simulink model "MLC_Aero_Simulink"  (R2018a)
settings: Solver=ode1  StartTime=0.0  StopTime=50  FixedStep=0.002  RelTol=1e-3  EnableMultiTasking=on
values from neighbouring files (symbols this model uses):
  pitch_amp = pi/6    (= 0.523598775598)    [lqr_controller.m]
  pitch_freq = 0.4    [lqr_controller.m]
  yaw_amp = pi/4    (= 0.785398163397)    [lqr_controller.m]
  yaw_freq = 0.5    [lqr_controller.m]
undefined symbols (not defined in the file or in its folder): HIL, qc_get_step_size
libraries: quarc_library x18, cstblocks x5
settings Model: SimulationMode=external  ExtModeTrigDuration=20000  Creator=MLevis  LastModifiedBy=Student
settings SolverCC: PositivePriorityOrder=on
settings DataIOCC: LimitDataPoints=on  SaveFormat=Array
settings OptimizationCC: LifeSpan=inf
settings DebuggingCC: SolverPrmCheckMsg=warning  SFUnexpectedBacktrackingDiag=warning  SFNoUnconditionalDefaultTransitionDiag=warning  SFExecutionAtInitializationDiag=none
settings HardwareCC: ProdBitPerPointer=32  ProdBitPerSizeT=32  ProdBitPerPtrDiffT=32  ProdLargestAtomicFloat=None  ProdIntDivRoundTo=Undefined  ProdEndianess=Unspecified  ProdWordSize=32  ProdHWDeviceType=32-bit Generic
settings ModelReferenceCC: PropagateSignalLabelsOutOfModel=off
settings RTWCC: SystemTargetFile=quarc_win64.tlc  TemplateMakefile=quarc_default_tmf  Description=QUARC Win64 Target
settings CodeAppCC: StateflowObjectComments=on
settings STFCustomTargetCC: TargetPreCompLibLocation=C:\PROGRA~3\QUARC\lib\2018a\win64\release  ConcurrentExecutionCompliant=on  GeneratePreprocessorConditionals=Disable all  SystemTargetFile=quarc_win64.tlc
settings GRTTargetCC: TargetPreCompLibLocation=C:\PROGRA~3\QUARC\lib\2018a\win64\release  TargetLangStandard=C89/C90 (ANSI)  ParMdlRefBuildCompliant=off  CompOptLevelCompliant=off  GeneratePreprocessorConditionals=Disable all  CombineOutputUpdateFcns=off  MatFileLogging=off  CPPClassGenCompliant=off  GRTInterface=on  UseToolchainInfoCompliant=off  ExtMode=on  ExtModeMexFile=quarc_comm
settings ConfigComp: CovMetricSettings=dw  CovHtmlReporting=on  CovSaveCumulativeToWorkspaceVar=on  CovSaveSingleToWorkspaceVar=on  CovExternalEMLEnable=off  CovSFcnEnable=off

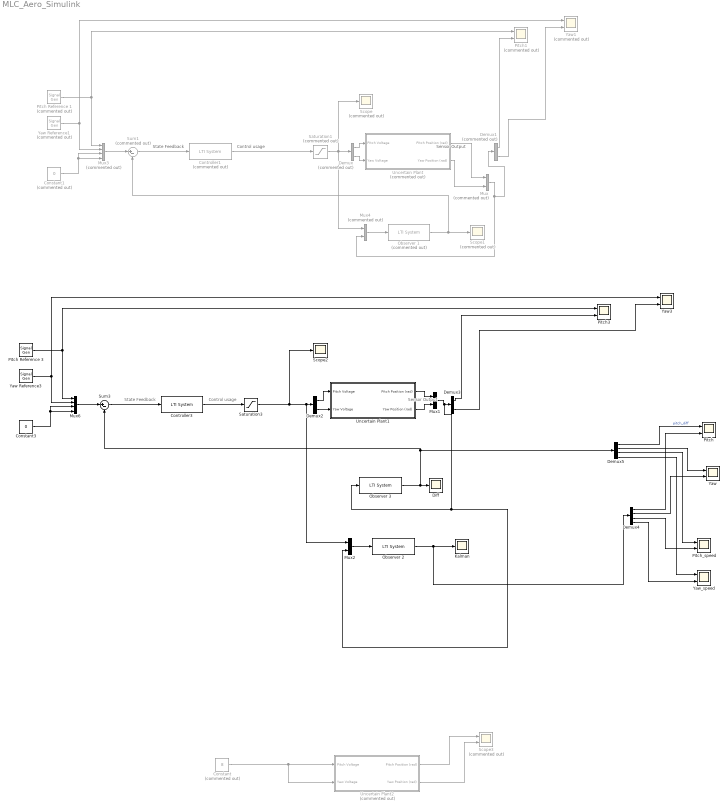
== system MLC_Aero_Simulink ==
  note: Sensor Output
  note: State Feedback
  note: Control usage
  note: Control usage
  note: Sensor Output
  note: State Feedback
  Constant : Constant  Commented=on  Value=8
  Constant1 : Constant  Commented=on  Value=0
  Constant3 : Constant  Value=0
  Controller1 : cstblocks/LTI System  Commented=on  sys=K  IC=[]
  Controller3 : cstblocks/LTI System  sys=K  IC=[]
  Demux : Demux  Commented=on  Outputs=2
  Demux1 : Demux  Commented=on  Outputs=2
  Demux2 : Demux  Outputs=2
  Demux3 : Demux  Outputs=2
  Demux4 : Demux
  Demux5 : Demux
  Diff : Scope
  "Kalman " : Scope
  Mux : Mux  Commented=on  Inputs=2
  Mux1 : Mux  Inputs=2
  Mux2 : Mux  Inputs=2
  Mux3 : Mux  Commented=on
  Mux4 : Mux  Commented=on  Inputs=2
  Mux6 : Mux
  Observer 1 : cstblocks/LTI System  Commented=on  sys=obs_sys_kalman  IC=[0.1,0.1,0,0]
  Observer 2 : cstblocks/LTI System  sys=obs_sys_kalman  IC=[0,0,0,0]
  Observer 3 : cstblocks/LTI System  sys=obs_sys_diff  IC=[]
  Pitch : Scope  NumInputPorts=2
  Pitch Reference 1 : SignalGenerator  Commented=on  WaveForm=square  Amplitude=pitch_amp  Frequency=pitch_freq  Units=rad/sec
  Pitch Reference 3 : SignalGenerator  WaveForm=square  Amplitude=pitch_amp  Frequency=pitch_freq  Units=rad/sec
  Pitch1 : Scope  Commented=on  NumInputPorts=2
  Pitch3 : Scope  NumInputPorts=2
  Pitch_speed : Scope  NumInputPorts=2
  Saturation1 : Saturate  Commented=on  UpperLimit=25  LowerLimit=-25
  Saturation3 : Saturate  UpperLimit=25  LowerLimit=-25
  Scope : Scope  Commented=on
  Scope1 : Scope  Commented=on
  Scope2 : Scope
  Scope3 : Scope  Commented=on  NumInputPorts=2
  Sum1 : Sum  Commented=on  Inputs=|+-
  Sum3 : Sum  Inputs=|+-
  Uncertain Plant : Subsystem  Commented=on
  Uncertain Plant1 : Subsystem
  Uncertain Plant2 : Subsystem  Commented=on
  Yaw : Scope  NumInputPorts=2
  Yaw Reference1 : SignalGenerator  Commented=on  WaveForm=square  Amplitude=yaw_amp  Frequency=yaw_freq  Units=rad/sec
  Yaw Reference3 : SignalGenerator  WaveForm=square  Amplitude=yaw_amp  Frequency=yaw_freq  Units=rad/sec
  Yaw1 : Scope  Commented=on  NumInputPorts=2
  Yaw3 : Scope  NumInputPorts=2
  Yaw_speed : Scope  NumInputPorts=2
  wires:
  Pitch Reference 1/1 -> Pitch1/1, Mux3/1
  Mux3/1 -> Sum1/1
  Constant1/1 -> Mux3/3, Mux3/4
  Controller1/1 -> Saturation1/1
  Yaw Reference1/1 -> Mux3/2, Yaw1/1
  Saturation1/1 -> Scope/1, Demux/1, Mux4/1
  Mux4/1 -> Observer 1/1
  Sum1/1 -> Controller1/1
  Observer 1/1 -> Sum1/2, Scope1/1
  Demux1/1 -> Pitch1/2
  Demux1/2 -> Yaw1/2
  Demux/1 -> Uncertain Plant/1(Pitch Voltage)
  Demux/2 -> Uncertain Plant/2(Yaw Voltage)
  Uncertain Plant/1(Pitch Position (rad)) -> Mux/1
  Uncertain Plant/2(Yaw Position (rad)) -> Mux/2
  Mux/1 -> Demux1/1, Mux4/2
  Yaw Reference3/1 -> Mux6/2, Yaw3/1
  Mux6/1 -> Sum3/1
  Demux3/2 -> Yaw3/2
  Demux3/1 -> Pitch3/2
  Pitch Reference 3/1 -> Pitch3/1, Mux6/1
  Controller3/1 -> Saturation3/1
  Constant3/1 -> Mux6/3, Mux6/4
  Sum3/1 -> Controller3/1
  Observer 3/1 -> Demux5/1, Sum3/2, Diff/1
  Saturation3/1 -> Scope2/1, Mux2/1, Demux2/1
  Demux2/1 -> Uncertain Plant1/1(Pitch Voltage)
  Demux2/2 -> Uncertain Plant1/2(Yaw Voltage)
  Uncertain Plant1/1(Pitch Position (rad)) -> Mux1/1
  Uncertain Plant1/2(Yaw Position (rad)) -> Mux1/2
  Mux1/1 -> Mux2/2, Observer 3/1, Demux3/1
  Observer 2/1 -> Demux4/1, "Kalman "/1
  Mux2/1 -> Observer 2/1
  Demux4/2 -> Yaw/2
  Demux4/1 -> Pitch/2
  Demux4/4 -> Yaw_speed/2
  Demux4/3 -> Pitch_speed/2
  Demux5/1 -> Pitch/1  "pitch_diff"
  Demux5/2 -> Yaw/1
  Demux5/3 -> Pitch_speed/1
  Demux5/4 -> Yaw_speed/1
  Constant/1 -> Uncertain Plant2/2(Yaw Voltage), Uncertain Plant2/1(Pitch Voltage)
  Uncertain Plant2/1(Pitch Position (rad)) -> Scope3/1
  Uncertain Plant2/2(Yaw Position (rad)) -> Scope3/2

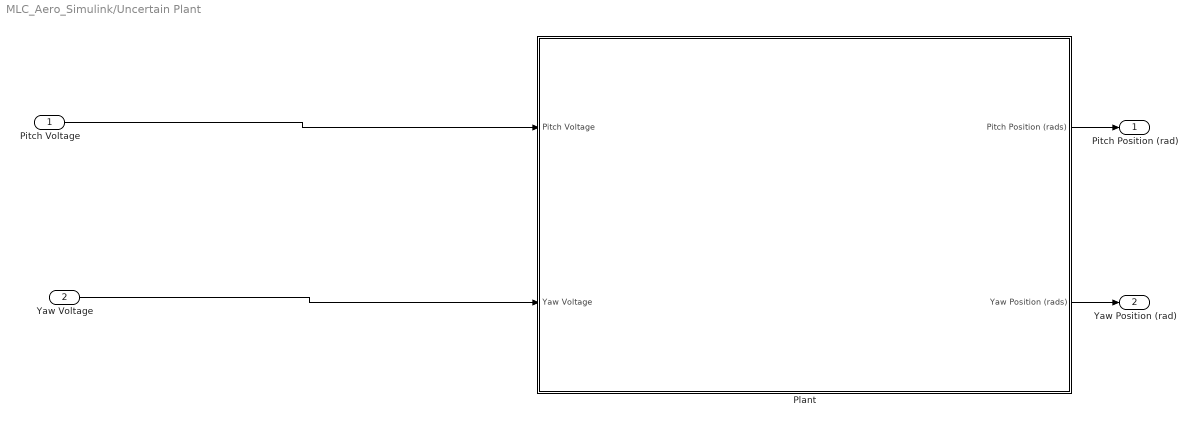
== system MLC_Aero_Simulink/Uncertain Plant ==
  Pitch Voltage : Inport
  Yaw Voltage : Inport  Port=2
  Plant : Subsystem
  Pitch Position (rad) : Outport
  Yaw Position (rad) : Outport  Port=2
  wires:
  Pitch Voltage/1 -> Plant/1(Pitch Voltage)
  Yaw Voltage/1 -> Plant/2(Yaw Voltage)
  Plant/1(Pitch Position (rads)) -> Pitch Position (rad)/1
  Plant/2(Yaw Position (rads)) -> Yaw Position (rad)/1

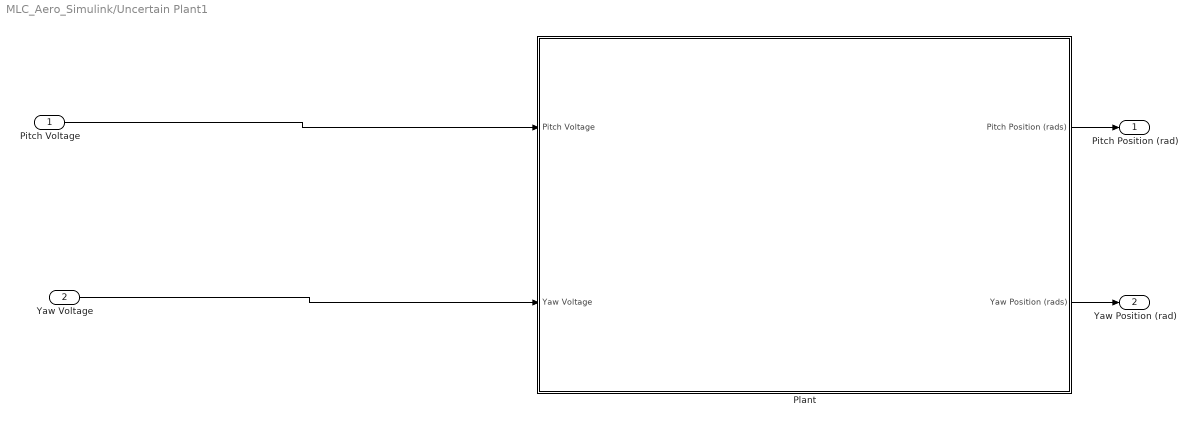
== system MLC_Aero_Simulink/Uncertain Plant1 ==
  Pitch Voltage : Inport
  Yaw Voltage : Inport  Port=2
  Plant : Subsystem
  Pitch Position (rad) : Outport
  Yaw Position (rad) : Outport  Port=2
  wires:
  Plant/2(Yaw Position (rads)) -> Yaw Position (rad)/1
  Plant/1(Pitch Position (rads)) -> Pitch Position (rad)/1
  Yaw Voltage/1 -> Plant/2(Yaw Voltage)
  Pitch Voltage/1 -> Plant/1(Pitch Voltage)

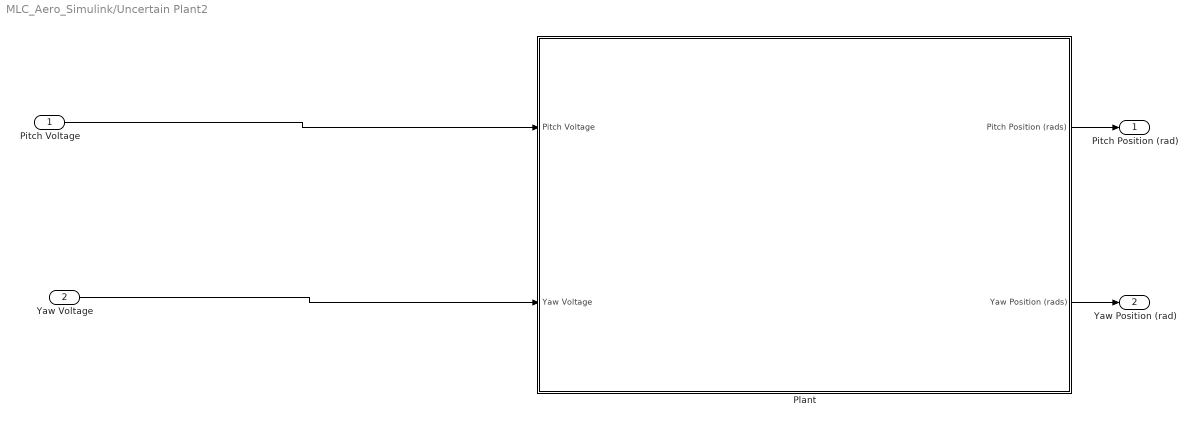
== system MLC_Aero_Simulink/Uncertain Plant2 ==
  Pitch Voltage : Inport
  Yaw Voltage : Inport  Port=2
  Plant : Subsystem
  Pitch Position (rad) : Outport
  Yaw Position (rad) : Outport  Port=2
  wires:
  Pitch Voltage/1 -> Plant/1(Pitch Voltage)
  Yaw Voltage/1 -> Plant/2(Yaw Voltage)
  Plant/1(Pitch Position (rads)) -> Pitch Position (rad)/1
  Plant/2(Yaw Position (rads)) -> Yaw Position (rad)/1

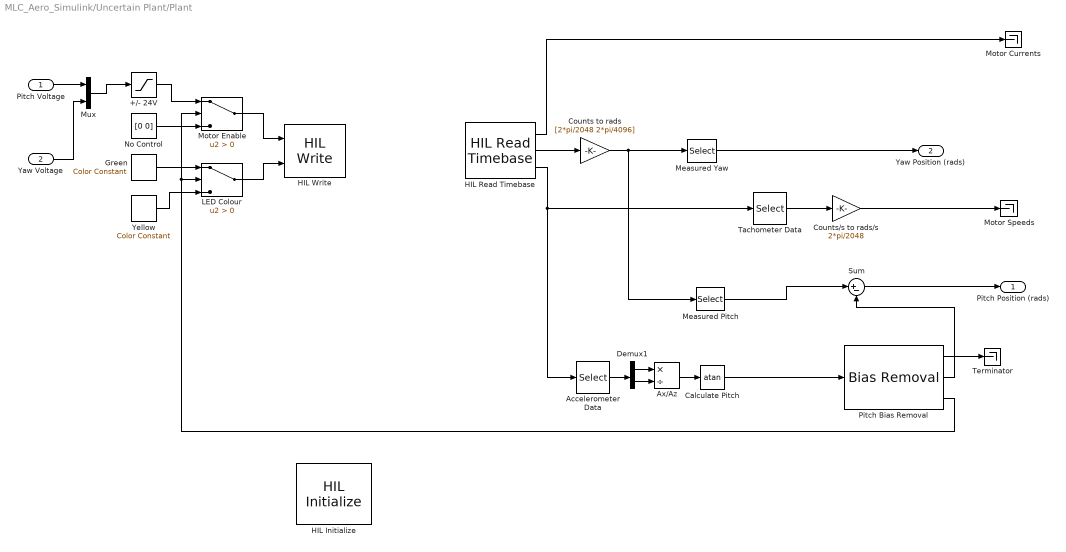
== system MLC_Aero_Simulink/Uncertain Plant/Plant ==
  Pitch Voltage : Inport
  Yaw Voltage : Inport  Port=2
  +/- 24V : Saturate  UpperLimit=24  LowerLimit=-24
  Accelerometer Data : Selector  InputPortWidth=4  IndexOptions=Index vector (dialog)  Indices=[1 2]  OutputSizes=1
  Ax/Az : Product  Inputs=*/
  Calculate Pitch : Trigonometry  Operator=atan
  Counts to rads : Gain  Gain=[2*pi/2048 2*pi/4096]
  Counts/s to rads/s : Gain  Gain=2*pi/2048
  Demux1 : Demux  Outputs=2
  Green : quarc_library/Sources/Signals/Color Constant  color=[0 1 0]
      settings: SourceProductName=QUARC Targets
  HIL Initialize : quarc_library/Data Acquisition/Generic/Configuration/HIL Initialize  Priority=-99  object_name=HIL-1  board_type=quanser_aero_usb  board_number=0  board_options=""  exclusive=off  active=off  hardware_clocks=[0]  clock_modes=[]  initial_clock_frequencies=[]  set_clock_params_at_start=off  set_clock_params_at_switch_in=off  set_clock_frequencies_at_start=off  set_clock_frequencies_at_switch_in=off  analog_input_channels=[0:1]  analog_input_configurations=0  analog_input_maximums=3  analog_input_minimums=-3  set_analog_input_params_at_start=off  set_analog_input_params_at_switch_in=off  analog_output_channels=[0:1]  analog_output_maximums=24  analog_output_minimums=-24  initial_analog_outputs=[0]  final_analog_outputs=[0]  watchdog_analog_outputs=[0]  set_analog_output_params_at_start=off  set_analog_output_params_at_switch_in=off  set_analog_outputs_at_start=on  set_analog_outputs_at_switch_in=off  set_analog_outputs_at_terminate=on  set_analog_outputs_at_switch_out=off  set_analog_outputs_on_watchdog=on  digital_input_channels=[]  digital_output_channels=[0:1]  digital_output_configuration=[]  initial_digital_outputs=[1]  final_digital_outputs=[0]  watchdog_digital_outputs=[0]  set_digital_output_params_at_start=off  set_digital_output_params_at_switch_in=off  set_digital_outputs_at_start=on  set_digital_outputs_at_switch_in=off  set_digital_outputs_at_terminate=on  set_digital_outputs_at_switch_out=off  set_digital_outputs_on_watchdog=on  encoder_channels=[0:3]  quadrature=[4]  encoder_filter_frequency=[]  initial_encoder_counts=[0]  set_encoder_params_at_start=off  set_encoder_params_at_switch_in=off  set_encoder_counts_at_start=on  set_encoder_counts_at_switch_in=off  pwm_channels=[]  pwm_modes=[]  pwm_frequency=[]  pwm_configuration=[]  pwm_alignment=[]  pwm_polarity=[]  pwm_leading_deadband=[]  pwm_trailing_deadband=[]  initial_pwm_outputs=[]  final_pwm_outputs=[]  watchdog_pwm_outputs=[]  set_pwm_params_at_start=off  set_pwm_params_at_switch_in=off  set_pwm_outputs_at_start=off  set_pwm_outputs_at_switch_in=off  set_pwm_outputs_at_terminate=off  set_pwm_outputs_at_switch_out=off  set_pwm_outputs_on_watchdog=off  other_output_channels=[11000:11002]  initial_other_outputs=[0 1 0]  final_other_outputs=[1 0 0]  watchdog_other_outputs=[0 0 1]  set_other_outputs_at_start=on  set_other_outputs_at_switch_in=off  set_other_outputs_at_terminate=on  set_other_outputs_at_switch_out=off  set_other_outputs_on_watchdog=on
  HIL Read Timebase : quarc_library/Data Acquisition/Generic/Timebases/HIL Read Timebase  object_name=HIL-1  clock=0  analog_channels=[0:1]  encoder_channels=[2:3]  digital_channels=[]  other_channels=[4000 4002 14000 14001]  samples_in_buffer=max(ceil(1/qc_get_step_size), 1)  active=on  vector_output=on  data_type_mode=Inherit via back propagation  encoder_data_type=double  digital_data_type=boolean
  HIL Write : quarc_library/Data Acquisition/Generic/Immediate I//O/HIL Write  object_name=HIL-1  analog_channels=[0:1]  pwm_channels=[]  digital_channels=[]  other_channels=[11000:11002]  sample_time=-1  active=off  vector_input=on
  LED Colour : Switch  Criteria=u2 > Threshold
  Measured Pitch : Selector  InputPortWidth=2  IndexOptions=Index vector (dialog)  Indices=[1]  OutputSizes=1
  Measured Yaw : Selector  InputPortWidth=2  IndexOptions=Index vector (dialog)  Indices=[2]  OutputSizes=1
  Motor Currents : Terminator
  Motor Enable : Switch  Criteria=u2 > Threshold
  Motor Speeds : Terminator
  Mux : Mux  Inputs=2
  No Control : Constant  Value=[0 0]
  Pitch Bias Removal : quarc_library/Discrete/Bias Removal  start_time=0  end_time=1  switch_id=0  sample_time=qc_get_step_size
      settings: SourceProductName=QUARC Targets
  Sum : Sum  Inputs=|+-
  Tachometer Data : Selector  InputPortWidth=4  IndexOptions=Index vector (dialog)  Indices=[3 4]  OutputSizes=1
  Terminator : Terminator
  Yellow : quarc_library/Sources/Signals/Color Constant  color=[1 0 0]
      settings: SourceProductName=QUARC Targets
  Pitch Position (rads) : Outport
  Yaw Position (rads) : Outport  Port=2
  wires:
  Pitch Bias Removal/3 -> Motor Enable/2, LED Colour/2
  +/- 24V/1 -> Motor Enable/1
  Motor Enable/1 -> HIL Write/1
  Green/1 -> LED Colour/1
  Yellow/1 -> LED Colour/3
  LED Colour/1 -> HIL Write/2
  No Control/1 -> Motor Enable/3
  Tachometer Data/1 -> Counts/s to rads/s/1
  Demux1/1 -> Ax/Az/1
  Demux1/2 -> Ax/Az/2
  HIL Read Timebase/2 -> Counts to rads/1
  Calculate Pitch/1 -> Pitch Bias Removal/1
  Counts/s to rads/s/1 -> Motor Speeds/1
  HIL Read Timebase/1 -> Motor Currents/1
  Accelerometer Data/1 -> Demux1/1
  HIL Read Timebase/3 -> Accelerometer Data/1, Tachometer Data/1
  Counts to rads/1 -> Measured Pitch/1, Measured Yaw/1
  Ax/Az/1 -> Calculate Pitch/1
  Pitch Bias Removal/2 -> Sum/2
  Pitch Voltage/1 -> Mux/1
  Yaw Voltage/1 -> Mux/2
  Mux/1 -> +/- 24V/1
  Pitch Bias Removal/1 -> Terminator/1
  Sum/1 -> Pitch Position (rads)/1
  Measured Pitch/1 -> Sum/1
  Measured Yaw/1 -> Yaw Position (rads)/1

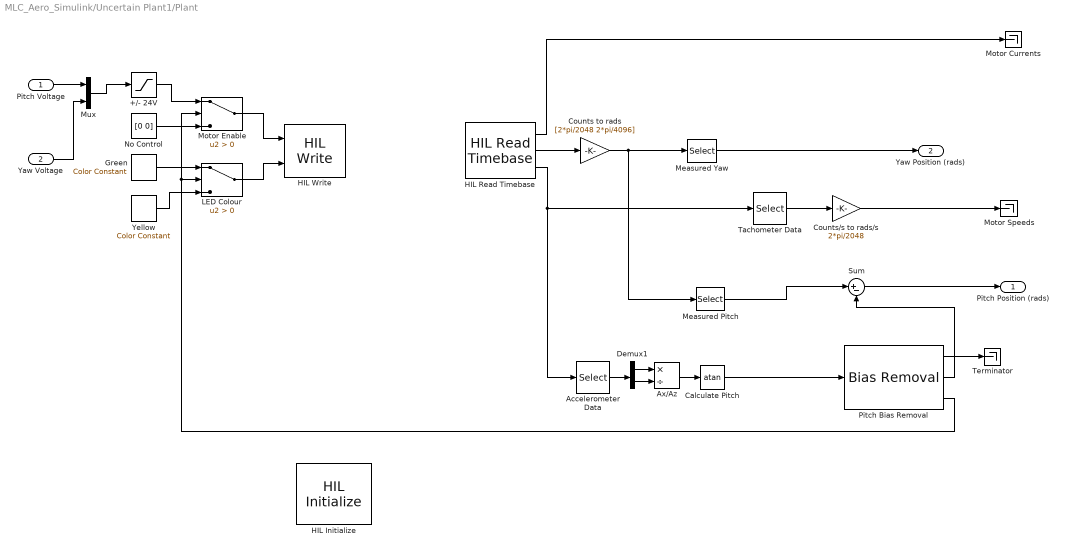
== system MLC_Aero_Simulink/Uncertain Plant1/Plant ==
  Pitch Voltage : Inport
  Yaw Voltage : Inport  Port=2
  +/- 24V : Saturate  UpperLimit=24  LowerLimit=-24
  Accelerometer Data : Selector  InputPortWidth=4  IndexOptions=Index vector (dialog)  Indices=[1 2]  OutputSizes=1
  Ax/Az : Product  Inputs=*/
  Calculate Pitch : Trigonometry  Operator=atan
  Counts to rads : Gain  Gain=[2*pi/2048 2*pi/4096]
  Counts/s to rads/s : Gain  Gain=2*pi/2048
  Demux1 : Demux  Outputs=2
  Green : quarc_library/Sources/Signals/Color Constant  color=[0 1 0]
      settings: SourceProductName=QUARC Targets
  HIL Initialize : quarc_library/Data Acquisition/Generic/Configuration/HIL Initialize  Priority=-99  object_name=HIL-1  board_type=quanser_aero_usb  board_number=0  board_options=""  exclusive=off  active=off  hardware_clocks=[0]  clock_modes=[]  initial_clock_frequencies=[]  set_clock_params_at_start=off  set_clock_params_at_switch_in=off  set_clock_frequencies_at_start=off  set_clock_frequencies_at_switch_in=off  analog_input_channels=[0:1]  analog_input_configurations=0  analog_input_maximums=3  analog_input_minimums=-3  set_analog_input_params_at_start=off  set_analog_input_params_at_switch_in=off  analog_output_channels=[0:1]  analog_output_maximums=24  analog_output_minimums=-24  initial_analog_outputs=[0]  final_analog_outputs=[0]  watchdog_analog_outputs=[0]  set_analog_output_params_at_start=off  set_analog_output_params_at_switch_in=off  set_analog_outputs_at_start=on  set_analog_outputs_at_switch_in=off  set_analog_outputs_at_terminate=on  set_analog_outputs_at_switch_out=off  set_analog_outputs_on_watchdog=on  digital_input_channels=[]  digital_output_channels=[0:1]  digital_output_configuration=[]  initial_digital_outputs=[1]  final_digital_outputs=[0]  watchdog_digital_outputs=[0]  set_digital_output_params_at_start=off  set_digital_output_params_at_switch_in=off  set_digital_outputs_at_start=on  set_digital_outputs_at_switch_in=off  set_digital_outputs_at_terminate=on  set_digital_outputs_at_switch_out=off  set_digital_outputs_on_watchdog=on  encoder_channels=[0:3]  quadrature=[4]  encoder_filter_frequency=[]  initial_encoder_counts=[0]  set_encoder_params_at_start=off  set_encoder_params_at_switch_in=off  set_encoder_counts_at_start=on  set_encoder_counts_at_switch_in=off  pwm_channels=[]  pwm_modes=[]  pwm_frequency=[]  pwm_configuration=[]  pwm_alignment=[]  pwm_polarity=[]  pwm_leading_deadband=[]  pwm_trailing_deadband=[]  initial_pwm_outputs=[]  final_pwm_outputs=[]  watchdog_pwm_outputs=[]  set_pwm_params_at_start=off  set_pwm_params_at_switch_in=off  set_pwm_outputs_at_start=off  set_pwm_outputs_at_switch_in=off  set_pwm_outputs_at_terminate=off  set_pwm_outputs_at_switch_out=off  set_pwm_outputs_on_watchdog=off  other_output_channels=[11000:11002]  initial_other_outputs=[0 1 0]  final_other_outputs=[1 0 0]  watchdog_other_outputs=[0 0 1]  set_other_outputs_at_start=on  set_other_outputs_at_switch_in=off  set_other_outputs_at_terminate=on  set_other_outputs_at_switch_out=off  set_other_outputs_on_watchdog=on
  HIL Read Timebase : quarc_library/Data Acquisition/Generic/Timebases/HIL Read Timebase  object_name=HIL-1  clock=0  analog_channels=[0:1]  encoder_channels=[2:3]  digital_channels=[]  other_channels=[4000 4002 14000 14001]  samples_in_buffer=max(ceil(1/qc_get_step_size), 1)  active=on  vector_output=on  data_type_mode=Inherit via back propagation  encoder_data_type=double  digital_data_type=boolean
  HIL Write : quarc_library/Data Acquisition/Generic/Immediate I//O/HIL Write  object_name=HIL-1  analog_channels=[0:1]  pwm_channels=[]  digital_channels=[]  other_channels=[11000:11002]  sample_time=-1  active=off  vector_input=on
  LED Colour : Switch  Criteria=u2 > Threshold
  Measured Pitch : Selector  InputPortWidth=2  IndexOptions=Index vector (dialog)  Indices=[1]  OutputSizes=1
  Measured Yaw : Selector  InputPortWidth=2  IndexOptions=Index vector (dialog)  Indices=[2]  OutputSizes=1
  Motor Currents : Terminator
  Motor Enable : Switch  Criteria=u2 > Threshold
  Motor Speeds : Terminator
  Mux : Mux  Inputs=2
  No Control : Constant  Value=[0 0]
  Pitch Bias Removal : quarc_library/Discrete/Bias Removal  start_time=0  end_time=1  switch_id=0  sample_time=qc_get_step_size
      settings: SourceProductName=QUARC Targets
  Sum : Sum  Inputs=|+-
  Tachometer Data : Selector  InputPortWidth=4  IndexOptions=Index vector (dialog)  Indices=[3 4]  OutputSizes=1
  Terminator : Terminator
  Yellow : quarc_library/Sources/Signals/Color Constant  color=[1 0 0]
      settings: SourceProductName=QUARC Targets
  Pitch Position (rads) : Outport
  Yaw Position (rads) : Outport  Port=2
  wires:
  Measured Yaw/1 -> Yaw Position (rads)/1
  Measured Pitch/1 -> Sum/1
  Sum/1 -> Pitch Position (rads)/1
  Pitch Bias Removal/1 -> Terminator/1
  Mux/1 -> +/- 24V/1
  Yaw Voltage/1 -> Mux/2
  Pitch Voltage/1 -> Mux/1
  Pitch Bias Removal/2 -> Sum/2
  Ax/Az/1 -> Calculate Pitch/1
  Counts to rads/1 -> Measured Yaw/1, Measured Pitch/1
  HIL Read Timebase/3 -> Tachometer Data/1, Accelerometer Data/1
  Accelerometer Data/1 -> Demux1/1
  HIL Read Timebase/1 -> Motor Currents/1
  Counts/s to rads/s/1 -> Motor Speeds/1
  Calculate Pitch/1 -> Pitch Bias Removal/1
  HIL Read Timebase/2 -> Counts to rads/1
  Demux1/2 -> Ax/Az/2
  Demux1/1 -> Ax/Az/1
  Tachometer Data/1 -> Counts/s to rads/s/1
  No Control/1 -> Motor Enable/3
  LED Colour/1 -> HIL Write/2
  Yellow/1 -> LED Colour/3
  Green/1 -> LED Colour/1
  Motor Enable/1 -> HIL Write/1
  +/- 24V/1 -> Motor Enable/1
  Pitch Bias Removal/3 -> LED Colour/2, Motor Enable/2

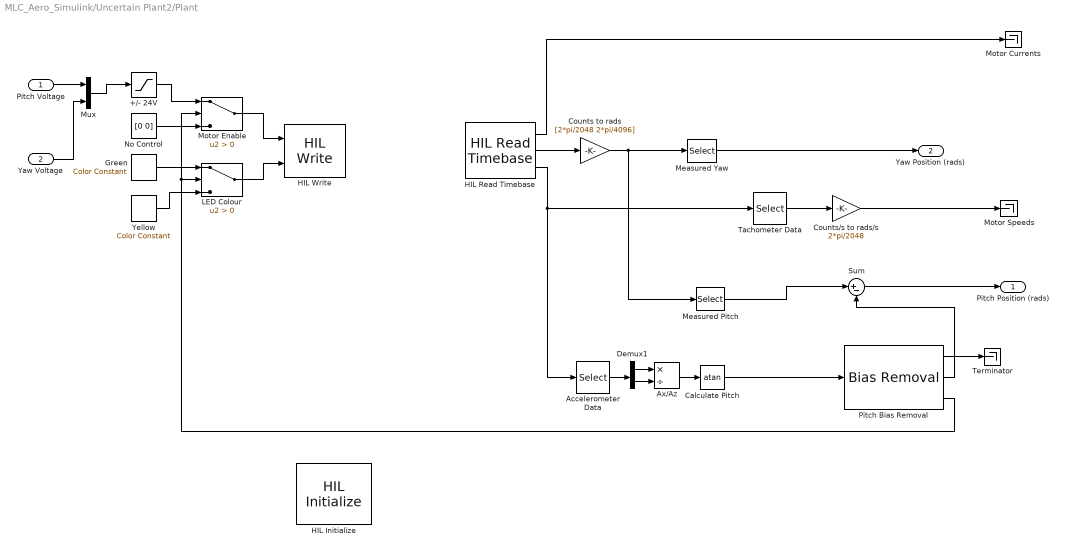
== system MLC_Aero_Simulink/Uncertain Plant2/Plant ==
  Pitch Voltage : Inport
  Yaw Voltage : Inport  Port=2
  +/- 24V : Saturate  UpperLimit=24  LowerLimit=-24
  Accelerometer Data : Selector  InputPortWidth=4  IndexOptions=Index vector (dialog)  Indices=[1 2]  OutputSizes=1
  Ax/Az : Product  Inputs=*/
  Calculate Pitch : Trigonometry  Operator=atan
  Counts to rads : Gain  Gain=[2*pi/2048 2*pi/4096]
  Counts/s to rads/s : Gain  Gain=2*pi/2048
  Demux1 : Demux  Outputs=2
  Green : quarc_library/Sources/Signals/Color Constant  color=[0 1 0]
      settings: SourceProductName=QUARC Targets
  HIL Initialize : quarc_library/Data Acquisition/Generic/Configuration/HIL Initialize  Priority=-99  object_name=HIL-1  board_type=quanser_aero_usb  board_number=0  board_options=""  exclusive=off  active=off  hardware_clocks=[0]  clock_modes=[]  initial_clock_frequencies=[]  set_clock_params_at_start=off  set_clock_params_at_switch_in=off  set_clock_frequencies_at_start=off  set_clock_frequencies_at_switch_in=off  analog_input_channels=[0:1]  analog_input_configurations=0  analog_input_maximums=3  analog_input_minimums=-3  set_analog_input_params_at_start=off  set_analog_input_params_at_switch_in=off  analog_output_channels=[0:1]  analog_output_maximums=24  analog_output_minimums=-24  initial_analog_outputs=[0]  final_analog_outputs=[0]  watchdog_analog_outputs=[0]  set_analog_output_params_at_start=off  set_analog_output_params_at_switch_in=off  set_analog_outputs_at_start=on  set_analog_outputs_at_switch_in=off  set_analog_outputs_at_terminate=on  set_analog_outputs_at_switch_out=off  set_analog_outputs_on_watchdog=on  digital_input_channels=[]  digital_output_channels=[0:1]  digital_output_configuration=[]  initial_digital_outputs=[1]  final_digital_outputs=[0]  watchdog_digital_outputs=[0]  set_digital_output_params_at_start=off  set_digital_output_params_at_switch_in=off  set_digital_outputs_at_start=on  set_digital_outputs_at_switch_in=off  set_digital_outputs_at_terminate=on  set_digital_outputs_at_switch_out=off  set_digital_outputs_on_watchdog=on  encoder_channels=[0:3]  quadrature=[4]  encoder_filter_frequency=[]  initial_encoder_counts=[0]  set_encoder_params_at_start=off  set_encoder_params_at_switch_in=off  set_encoder_counts_at_start=on  set_encoder_counts_at_switch_in=off  pwm_channels=[]  pwm_modes=[]  pwm_frequency=[]  pwm_configuration=[]  pwm_alignment=[]  pwm_polarity=[]  pwm_leading_deadband=[]  pwm_trailing_deadband=[]  initial_pwm_outputs=[]  final_pwm_outputs=[]  watchdog_pwm_outputs=[]  set_pwm_params_at_start=off  set_pwm_params_at_switch_in=off  set_pwm_outputs_at_start=off  set_pwm_outputs_at_switch_in=off  set_pwm_outputs_at_terminate=off  set_pwm_outputs_at_switch_out=off  set_pwm_outputs_on_watchdog=off  other_output_channels=[11000:11002]  initial_other_outputs=[0 1 0]  final_other_outputs=[1 0 0]  watchdog_other_outputs=[0 0 1]  set_other_outputs_at_start=on  set_other_outputs_at_switch_in=off  set_other_outputs_at_terminate=on  set_other_outputs_at_switch_out=off  set_other_outputs_on_watchdog=on
  HIL Read Timebase : quarc_library/Data Acquisition/Generic/Timebases/HIL Read Timebase  object_name=HIL-1  clock=0  analog_channels=[0:1]  encoder_channels=[2:3]  digital_channels=[]  other_channels=[4000 4002 14000 14001]  samples_in_buffer=max(ceil(1/qc_get_step_size), 1)  active=on  vector_output=on  data_type_mode=Inherit via back propagation  encoder_data_type=double  digital_data_type=boolean
  HIL Write : quarc_library/Data Acquisition/Generic/Immediate I//O/HIL Write  object_name=HIL-1  analog_channels=[0:1]  pwm_channels=[]  digital_channels=[]  other_channels=[11000:11002]  sample_time=-1  active=off  vector_input=on
  LED Colour : Switch  Criteria=u2 > Threshold
  Measured Pitch : Selector  InputPortWidth=2  IndexOptions=Index vector (dialog)  Indices=[1]  OutputSizes=1
  Measured Yaw : Selector  InputPortWidth=2  IndexOptions=Index vector (dialog)  Indices=[2]  OutputSizes=1
  Motor Currents : Terminator
  Motor Enable : Switch  Criteria=u2 > Threshold
  Motor Speeds : Terminator
  Mux : Mux  Inputs=2
  No Control : Constant  Value=[0 0]
  Pitch Bias Removal : quarc_library/Discrete/Bias Removal  start_time=0  end_time=1  switch_id=0  sample_time=qc_get_step_size
      settings: SourceProductName=QUARC Targets
  Sum : Sum  Inputs=|+-
  Tachometer Data : Selector  InputPortWidth=4  IndexOptions=Index vector (dialog)  Indices=[3 4]  OutputSizes=1
  Terminator : Terminator
  Yellow : quarc_library/Sources/Signals/Color Constant  color=[1 0 0]
      settings: SourceProductName=QUARC Targets
  Pitch Position (rads) : Outport
  Yaw Position (rads) : Outport  Port=2
  wires:
  Pitch Bias Removal/3 -> Motor Enable/2, LED Colour/2
  +/- 24V/1 -> Motor Enable/1
  Motor Enable/1 -> HIL Write/1
  Green/1 -> LED Colour/1
  Yellow/1 -> LED Colour/3
  LED Colour/1 -> HIL Write/2
  No Control/1 -> Motor Enable/3
  Tachometer Data/1 -> Counts/s to rads/s/1
  Demux1/1 -> Ax/Az/1
  Demux1/2 -> Ax/Az/2
  HIL Read Timebase/2 -> Counts to rads/1
  Calculate Pitch/1 -> Pitch Bias Removal/1
  Counts/s to rads/s/1 -> Motor Speeds/1
  HIL Read Timebase/1 -> Motor Currents/1
  Accelerometer Data/1 -> Demux1/1
  HIL Read Timebase/3 -> Accelerometer Data/1, Tachometer Data/1
  Counts to rads/1 -> Measured Pitch/1, Measured Yaw/1
  Ax/Az/1 -> Calculate Pitch/1
  Pitch Bias Removal/2 -> Sum/2
  Pitch Voltage/1 -> Mux/1
  Yaw Voltage/1 -> Mux/2
  Mux/1 -> +/- 24V/1
  Pitch Bias Removal/1 -> Terminator/1
  Sum/1 -> Pitch Position (rads)/1
  Measured Pitch/1 -> Sum/1
  Measured Yaw/1 -> Yaw Position (rads)/1
